simulink model "Lab3_part2"  (R2025b)
settings: Solver=VariableStepAuto  StartTime=0.0  StopTime=2  RelTol=1e-3
values from neighbouring files (symbols this model uses):
  c = 2e-6    (= 2e-06)    [Lab3_part3.m]
  Rth_cl = (r3*r2)/(r3+r2)    (= 20000)    [Lab3_part3.m]
  Rth_op = (r2+r1)*r3/(r1+r2+r3)    (= 24000)    [Lab3_part3.m]
  Vth_cl = Vs*r3/(r3+r2)    (= 8)    [Lab3_part3.m]
  Vth_op = r3*Vs/(r1+r2+r3)    (= 7.2)    [Lab3_part3.m]
settings Model: Creator=Noah  LastModifiedBy=Noah

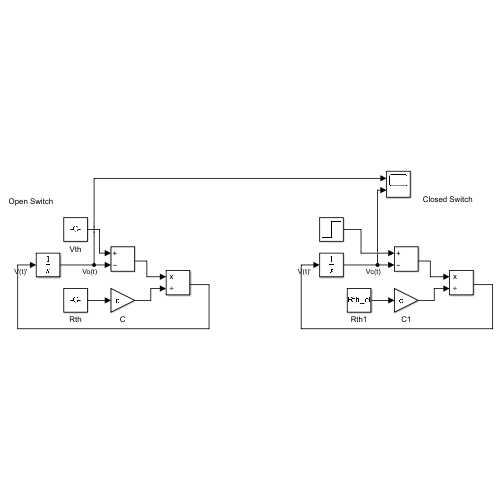
[thumbnail: Simulink's stored preview of the top-level diagram]
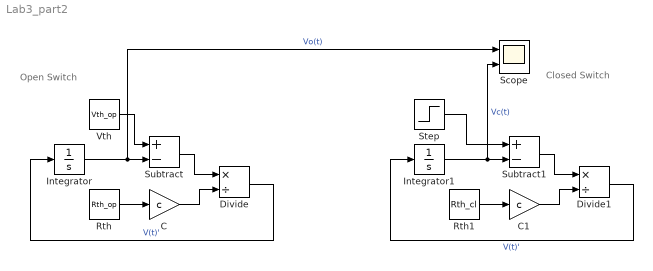
== system Lab3_part2 ==
  note: Closed Switch
  note: Open Switch
  C : Gain  Gain=c
  C1 : Gain  Gain=c
  Divide : Product  Inputs=*/
  Divide1 : Product  Inputs=*/
  Integrator : Integrator
  Integrator1 : Integrator  InitialCondition=7.2
  Rth : Constant  Value=Rth_op
  Rth1 : Constant  Value=Rth_cl
  Scope : Scope  NumInputPorts=2
      settings: ActiveDisplayYMinimum=-1.0286969652083249  ActiveDisplayYMaximum=9.4717522095774171
  Step : Step  Before=7.2  After=Vth_cl  SampleTime=0
  Subtract : Sum  Inputs=+-
  Subtract1 : Sum  Inputs=+-
  Vth : Constant  Value=Vth_op
  wires:
  Integrator/1 -> Scope/1, Subtract/2  "Vo(t)"
  Vth/1 -> Subtract/1
  Divide/1 -> Integrator/1  "V(t)'"
  Subtract/1 -> Divide/1
  C/1 -> Divide/2
  Rth/1 -> C/1
  Rth1/1 -> C1/1
  C1/1 -> Divide1/2
  Subtract1/1 -> Divide1/1
  Integrator1/1 -> Scope/2, Subtract1/2  "Vc(t)"
  Step/1 -> Subtract1/1
  Divide1/1 -> Integrator1/1  "V(t)'"
